simulink model "SimulinkOpenLoop"  (R2018b)
settings: Solver=VariableStepAuto  StartTime=0.0  StopTime=0.3  RelTol=1e-3
settings Model: Creator=victo  LastModifiedBy=victo

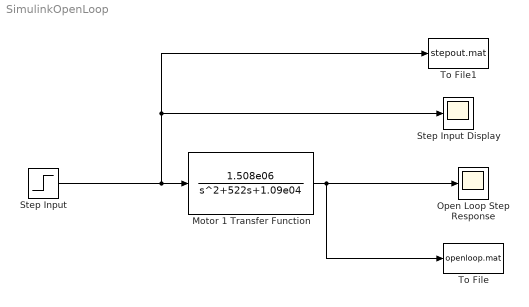
== system SimulinkOpenLoop ==
  Motor 1 Transfer Function : TransferFcn  Numerator=[1.508e06]  Denominator=[1 522 1.09e04]
  Open Loop Step Response : Scope
  Step Input : Step  Time=0  SampleTime=0.01
  Step Input Display : Scope
  To File : ToFile  Filename=openloop.mat  SaveFormat=Timeseries
  To File1 : ToFile  Filename=stepout.mat  SaveFormat=Timeseries
  wires:
  Step Input/1 -> To File1/1, Step Input Display/1, Motor 1 Transfer Function/1
  Motor 1 Transfer Function/1 -> To File/1, Open Loop Step Response/1
